simulink model "NewPVSys"  (R2024b)
settings: Solver=VariableStepAuto  StartTime=0.0  StopTime=10  RelTol=1e-3
undefined symbols (not defined in the file): Acid, Lead
libraries: spsSeriesRLCBranchLib x5, spsMosfetLib x3, spsCurrentMeasurementLib x2, spsVoltageMeasurementLib x2, spsPWMGeneratorDCDCLib x1, spsBatteryLib x1, spsDiodeLib x1, spsPVArrayLib x1, sps_lib x1
settings Model: Creator=joshbenner  LastModifiedBy=joshbenner
settings SolverCC: ZeroCrossAlgorithm=Adaptive
settings DebuggingCC: IgnoredZcDiagnostic=none

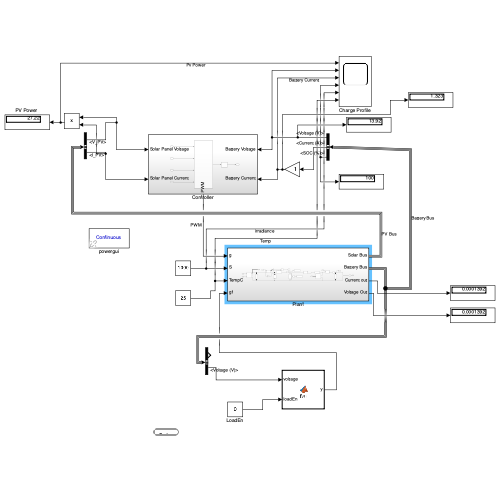
[thumbnail: Simulink's stored preview of the top-level diagram]
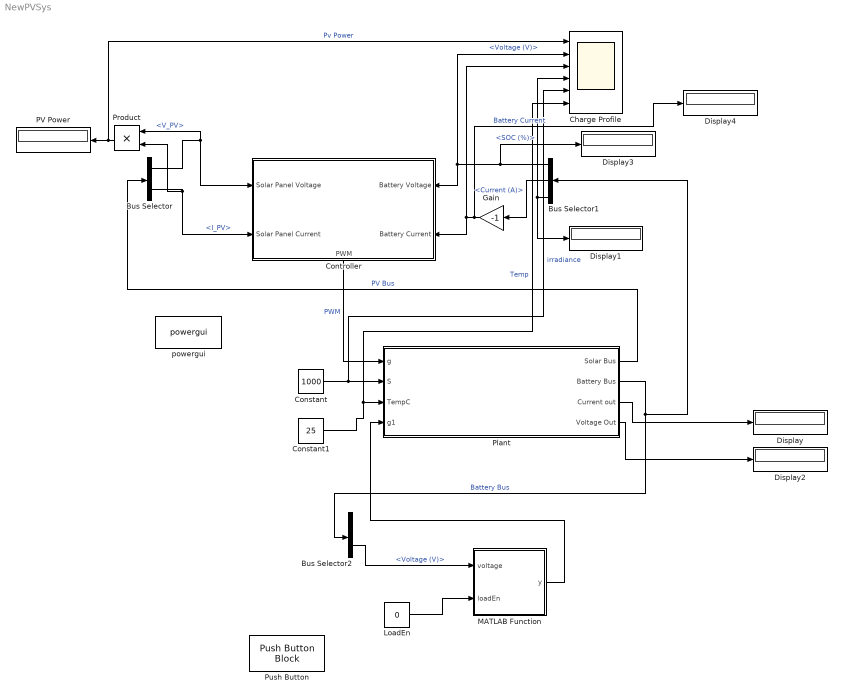
== system NewPVSys ==
  Bus Selector : BusSelector  OutputSignals=V_PV,I_PV
  Bus Selector1 : BusSelector  OutputSignals=Voltage (V),Current (A),SOC (%)
  Bus Selector2 : BusSelector  OutputSignals=Current (A),Voltage (V)
  Charge Profile : Scope  NumInputPorts=6
  Constant : Constant  Value=1000
  Constant1 : Constant  Value=25
  Controller : Subsystem
      settings: PortSchema="{\"entries\":[{\"content\":{\"sides\":[{\"content\":{\"connectorIds\":[\"In1\",\"In2\"]},\"type\":\"ConnectorPlacement.EquallySpacedRectSide\",\"uuid\":\"78124681-fbdc-4ce3-87f1-2df76917b9c7\"},{\"content\":{\"connectorIds\":[\"In3\",\"In4\"],\"side\":\"RIGHT\"},\"type\":\"ConnectorPlacement.EquallySpacedRectSide\",\"uuid\":\"c509d85d-9af4-46f5-94e8-4dea312fb1cd\"},{\"content\":{\"side\":\"TOP\"},\"type\":\"ConnectorPlacement.EquallySpacedRectSide\",\"uuid\":\"f654d0a5-48ca-4eb4-9ada-268228990754\"},{\"content\":{\"connectorIds\":[\"Out1\"],\"side\":\"BOTTOM\"},\"type\":\"ConnectorPlacement.EquallySpacedRectSide\",\"uuid\":\"ac5bad5c-0713-40be-a949-9f60af8c8d45\"}]},\"type\":\"ConnectorPlacement.EquallySpacedConnector\",\"uuid\":\"cd6d46ac-54d3-477c-b449-face08e3d569\"}],\"packageUris\":[\"http://schema.mathworks.com/mf0/Connector/R2020b\"],\"version\":\"1.0\"}"
  Display{,1..4} (5 alike) : Display
  Gain : Gain  Gain=-1
  LoadEn : Constant  Value=0
  MATLAB Function : MATLAB Function  TreatAsAtomicUnit=on
  "PV Power " : Display
  Plant : Subsystem
  Product : Product
  Push Button : PushButtonBlock  OffValue=0.000000
  powergui : sps_lib/powergui  Priority=1  SimulationMode=Continuous  SampleTime=50e-6  frequency=60  Iterations=50  frequencyindice=0  Pbase=100e6  ErrMax=1e-4  UnitsV=kV  UnitsW=MW  buscounter=0  FunctionMessages=off  echomessages=off  EnableUseOfTLC=off  CurrentSourceSwitches=off  DisableSnubberDevices=off  DisableRonSwitches=off  DisableVfSwitches=off  DisplayEquations=off  AutomaticDiscreteSolvers=off  SolverType=Tustin/Backward Euler (TBE)  Interpol=off  ExternalGateDelay=off  methode=off  Ts=100  x0status=blocks  SPID=on  SwTol=0  HookPort=off  NonlinearTolerance=1e-4  nMaxIteration=100  ContinueOnMaxIteration=off  RestoreLinks=warning  ResistiveCurrentMeasurement=off  Frange=[0:2:500]  Ylog=off  Xlog=on  ShowGrid=off  save=off  variable=ZData  structure=0  ZoomFFT=off  StartTime=0.0  cycles=1  DisplayStyle=1  fundamental=60  FreqAxis=off  MaxFrequency=1000  frequencyindicesteady=1  RmsSteady=1  display=off
  wires:
  Bus Selector/1 -> Product/1, Controller/1(Solar Panel Voltage)  "<V_PV>"
  Bus Selector/2 -> Product/2, Controller/2(Solar Panel Current)  "<I_PV>"
  Product/1 -> Charge Profile/1, "PV Power "/1  "Pv Power"
  Bus Selector1/1 -> Display3/1, Charge Profile/2, Controller/3(Battery Voltage)  "<Voltage (V)>"
  Bus Selector1/2 -> Gain/1  "<Current (A)>"
  Gain/1 -> Display4/1, Charge Profile/3, Controller/4(Battery Current)  "Battery Current"
  Bus Selector1/3 -> Display1/1, Charge Profile/4  "<SOC (%)>"
  Controller/1(PWM) -> Plant/1(g)  "PWM"
  Constant/1 -> Charge Profile/5, Plant/2(S)  "irradiance"
  Constant1/1 -> Charge Profile/6, Plant/3(TempC)  "Temp"
  Plant/1(Solar Bus) -> Bus Selector/1  "PV Bus"
  Plant/2(Battery Bus) -> Bus Selector2/1, Bus Selector1/1  "Battery Bus"
  MATLAB Function/1(y) -> Plant/4(g1)
  Bus Selector2/2 -> MATLAB Function/1(voltage)  "<Voltage (V)>"
  Plant/3(Current out) -> Display/1
  Plant/4(Voltage Out) -> Display2/1
  LoadEn/1 -> MATLAB Function/2(loadEn)

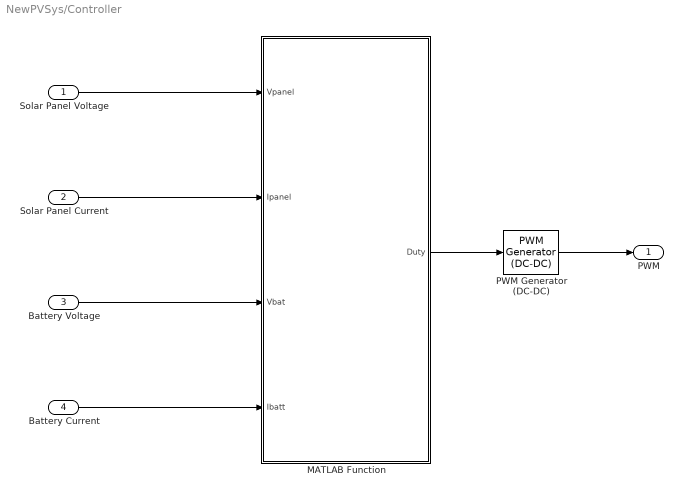
== system NewPVSys/Controller ==
  Solar Panel Voltage : Inport
  Solar Panel Current : Inport  Port=2
  Battery Voltage : Inport  Port=3
  Battery Current : Inport  Port=4
  MATLAB Function : MATLAB Function  TreatAsAtomicUnit=on
  PWM Generator (DC-DC) : spsPWMGeneratorDCDCLib/PWM Generator (DC-DC)  Fsw=100e3  Ts=0
  PWM : Outport
  wires:
  Solar Panel Voltage/1 -> MATLAB Function/1(Vpanel)
  Solar Panel Current/1 -> MATLAB Function/2(Ipanel)
  Battery Voltage/1 -> MATLAB Function/3(Vbat)
  Battery Current/1 -> MATLAB Function/4(Ibatt)
  MATLAB Function/1(Duty) -> PWM Generator (DC-DC)/1
  PWM Generator (DC-DC)/1 -> PWM/1

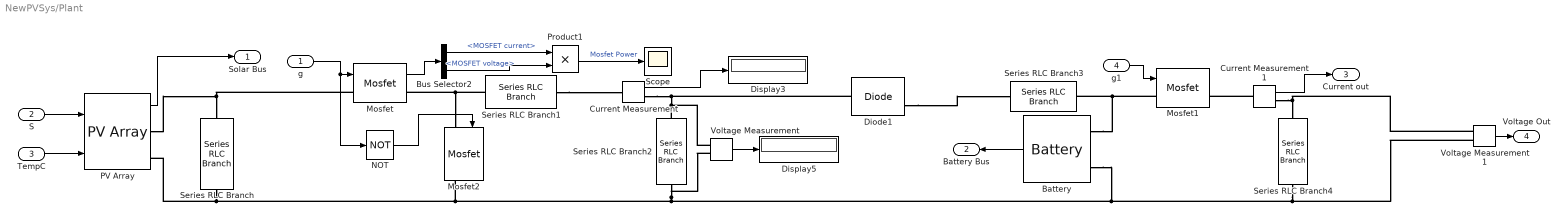
== system NewPVSys/Plant ==
  g : Inport
  S : Inport  Port=2
  TempC : Inport  Port=3
  g1 : Inport  Port=4
  Battery : spsBatteryLib/Battery  BatType=Lead-Acid  NomV=12  NomQ=5  SOC=100  Batt_Tr=1  PresetModel=on  MaxQ=5.2083  MinV=9  FullV=13.0658  Dis_rate=1  R=0.024  Normal_OP=1.5514  expZone="[12.2171    0.0166667]"
  Bus Selector2 : BusSelector  OutputSignals=MOSFET current,MOSFET voltage
  Current Measurement : spsCurrentMeasurementLib/Current Measurement  PhasorSimulation=off  OutputType=Complex  PSBequivalent=0
  Current Measurement1 : spsCurrentMeasurementLib/Current Measurement  PhasorSimulation=off  OutputType=Complex  PSBequivalent=0
  Diode1 : spsDiodeLib/Diode  Ron=0.001  Lon=0  Vf=0.8  IC=0  UseSnubber=0  Rs=500  Cs=250e-9  Measurements=on
  Display3 : Display
  Display5 : Display
  Mosfet : spsMosfetLib/Mosfet  Ron=0.1  Lon=0  Rd=0.01  Vfd=0  IC=0  Rs=1e5  Cs=inf  Measurements=on
  Mosfet1 : spsMosfetLib/Mosfet  Ron=0.1  Lon=0  Rd=0.01  Vfd=0  IC=0  Rs=1e5  Cs=inf  Measurements=on
  Mosfet2 : spsMosfetLib/Mosfet  Ron=0.1  Lon=0  Rd=0.01  Vfd=0  IC=0  Rs=1e5  Cs=inf  Measurements=on
  NOT : Logic  Operator=NOT  IconShape=distinctive  AllPortsSameDT=off  OutDataTypeStr=boolean
  PV Array : spsPVArrayLib/PV Array  Npar=1  Nser=1  PlotType=one module @ 25 deg.C & specified irradiances  S_vec="[ 1000  500  100 ]"  Temp_C_vec="[ 45 25  ]"  ModuleName=User-defined  PlotWhenSelected=off  Pm=52.92  Ncell=60  Voc=22.41  Isc=2.96  Vm=18  Im=2.94  beta_Voc_pc=-0.36099  alpha_Isc_pc=0.102  beta_Voc=-0.080898  alpha_Isc=0.0030192  IL=3.059  I0=1.116e-10  nI=0.6049  Rsh=6114.4954  Rs=0.58017  RobustModel=off  RobustCellTemperature=313.3991  BAL=on  Tc=1e-6  Tfilter=5e-5
  Product1 : Product
  Scope : Scope
  Series RLC Branch : spsSeriesRLCBranchLib/Series RLC Branch  LConnTagsString=__new0  RConnTagsString=__new0  BranchType=C  Resistance=.0001  Inductance=1e-3  SetiL0=off  InitialCurrent=0  Capacitance=1000e-6  Setx0=off  InitialVoltage=0  Measurements=None
  Series RLC Branch1 : spsSeriesRLCBranchLib/Series RLC Branch  LConnTagsString=__new0  RConnTagsString=__new0  BranchType=L  Resistance=.0001  Inductance=320e-3  SetiL0=off  InitialCurrent=0  Capacitance=1000e-6  Setx0=off  InitialVoltage=0  Measurements=None
  Series RLC Branch2 : spsSeriesRLCBranchLib/Series RLC Branch  LConnTagsString=__new0  RConnTagsString=__new0  BranchType=C  Resistance=.0001  Inductance=1e-3  SetiL0=off  InitialCurrent=0  Capacitance=20e-6  Setx0=off  InitialVoltage=0  Measurements=None
  Series RLC Branch3 : spsSeriesRLCBranchLib/Series RLC Branch  LConnTagsString=__new0  RConnTagsString=__new0  BranchType=R  Resistance=.0001  Inductance=1e-3  SetiL0=off  InitialCurrent=0  Capacitance=20e-6  Setx0=off  InitialVoltage=0  Measurements=None
  Series RLC Branch4 : spsSeriesRLCBranchLib/Series RLC Branch  LConnTagsString=__new0  RConnTagsString=__new0  BranchType=R  Resistance=1  Inductance=1e-3  SetiL0=off  InitialCurrent=0  Capacitance=20e-6  Setx0=off  InitialVoltage=0  Measurements=None
  Voltage Measurement : spsVoltageMeasurementLib/Voltage Measurement  PhasorSimulation=off  OutputType=Complex  PSBequivalent=0
  Voltage Measurement1 : spsVoltageMeasurementLib/Voltage Measurement  PhasorSimulation=off  OutputType=Complex  PSBequivalent=0
  Solar Bus : Outport
  Battery Bus : Outport  Port=2
  Current out : Outport  Port=3
  Voltage Out : Outport  Port=4
  wires:
  Battery/1 -> Battery Bus/1
  TempC/1 -> PV Array/2
  Bus Selector2/2 -> Product1/2  "<MOSFET voltage>"
  Product1/1 -> Scope/1  "Mosfet Power"
  Bus Selector2/1 -> Product1/1  "<MOSFET current>"
  S/1 -> PV Array/1
  Voltage Measurement/1 -> Display5/1
  PV Array/1 -> Solar Bus/1
  Current Measurement/1 -> Display3/1
  Mosfet/1 -> Bus Selector2/1
  g1/1 -> Mosfet1/1
  Current Measurement1/1 -> Current out/1
  Voltage Measurement1/1 -> Voltage Out/1
  g/1 -> NOT/1, Mosfet/1
  NOT/1 -> Mosfet2/1
  connections:
  Mosfet/LConn1 -- PV Array/RConn1 -- Series RLC Branch/LConn1
  Series RLC Branch1/RConn1 -- Current Measurement/LConn1
  Battery/LConn1 -- Mosfet1/LConn1 -- Series RLC Branch3/RConn1
  Series RLC Branch2/LConn1 -- Current Measurement/RConn1 -- Diode1/LConn1 -- Voltage Measurement/LConn1
  Series RLC Branch2/RConn1 -- Voltage Measurement/LConn2 -- Voltage Measurement1/LConn2 -- Series RLC Branch4/RConn1 -- Battery/LConn2 -- Series RLC Branch/RConn1 -- PV Array/RConn2 -- Mosfet2/RConn1
  Series RLC Branch1/LConn1 -- Mosfet/RConn1 -- Mosfet2/LConn1
  Voltage Measurement1/LConn1 -- Current Measurement1/RConn1 -- Series RLC Branch4/LConn1
  Current Measurement1/LConn1 -- Mosfet1/RConn1
  Diode1/RConn1 -- Series RLC Branch3/LConn1

== matlab function NewPVSys/MATLAB Function ==
  data: voltage input; y output; loadEn input
function y = fcn(voltage, loadEn)
if((voltage<11) || (loadEn==0 )) 
y=0;
else
    y=1; 
end

== matlab function NewPVSys/Controller/MATLAB Function ==
  settings: updateMethod=DISCRETE
  data: Vpanel input; Duty output; Ipanel input; Vbat input; Ibatt input
function Duty = MPPT_BMS_CurrentMode(Vpanel, Ipanel, Vbat, Ibatt)
% Combined MPPT + Charge-Current Limit using battery current feedback
% Now supports voltage-dependent Imax.

%% --- Persistent variables ---
persistent D MPPT_Duty V_old I_old freeze_MPPT

if isempty(D);            D = 0.5;        end
if isempty(MPPT_Duty);    MPPT_Duty = 0.5; end
if isempty(V_old);        V_old = Vpanel; end
if isempty(I_old);        I_old = Ipanel; end
if isempty(freeze_MPPT);  freeze_MPPT = false; end

%% --- PARAMETERS ---
DeltaD_MPPT    = 0.0005;  % Slow MPPT step
Kp_current     = 0.02;    % Fast current loop gain
MPPT_min_duty  = 0.05;

%% --- 1. COMPUTE VOLTAGE-DEPENDENT CHARGE CURRENT LIMIT ----
I_max = CurrentLimitFromVoltage(Vbat);

%% === 2. CURRENT-LIMIT LOOP (FAST, MASTER CONTROL) ===
I_error = I_max - Ibatt;

% Proportional control for current
D = D + Kp_current * I_error;

% Clamp fast-loop output
D = min(max(D, 0), 1);

%% Freeze MPPT when approaching current limit
if Ibatt > (0.98 * I_max)
    freeze_MPPT = true;
else
    freeze_MPPT = false;
end

%% === 3. MPPT LOOP (SLOW) ===
if ~freeze_MPPT
    Pnew = Vpanel * Ipanel;
    Pold = V_old * I_old;
    dP = Pnew - Pold;
    dV = Vpanel - V_old;

    % P&O logic for a buck converter
    if dP > 0
        if dV > 0
            MPPT_Duty = MPPT_Duty - DeltaD_MPPT;
        else
            MPPT_Duty = MPPT_Duty + DeltaD_MPPT;
        end
    elseif dP < 0
        if dV > 0
            MPPT_Duty = MPPT_Duty + DeltaD_MPPT;
        else
            MPPT_Duty = MPPT_Duty - DeltaD_MPPT;
        end
    end

    MPPT_Duty = min(max(MPPT_Duty, MPPT_min_duty), 1);
end

% Update PV memory
V_old = Vpanel;
I_old = Ipanel;

%% === 4. FINAL DUTY SELECTION ===
Duty = min(D, MPPT_Duty);

end

%% -----------------------------------------------------------
%% VOLTAGE-DEPENDENT CURRENT LIMIT FUNCTION
%% -----------------------------------------------------------
function Imax = CurrentLimitFromVoltage(Vbat)
% Customize these to your battery:
V_float      = 13.6;   % float transition voltage
V_absorb_end = 14.2;   % end of absorption
I_bulk       = 1.9;    % full bulk charge current
I_float      = 0.8;    % float charge current

if Vbat <= V_float
    % Bulk region → full current
    Imax = I_bulk;

elseif Vbat >= V_absorb_end
    % Float region → float current
    Imax = I_float;

else
    % Absorption region → linearly taper between I_bulk and I_float
    ratio = (Vbat - V_float) / (V_absorb_end - V_float);
    Imax = I_bulk - ratio * (I_bulk - I_float);
end
end
